simulink model "Final_3"  (R2022b)
settings: Solver=VariableStepAuto  StartTime=0.0  StopTime=20  RelTol=1e-3
libraries: cstblocks x22
settings Model: Creator=asus  LastModifiedBy=asus

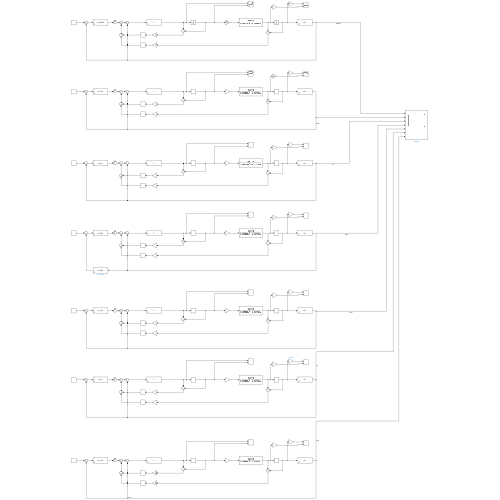
[thumbnail: Simulink's stored preview of the top-level diagram]
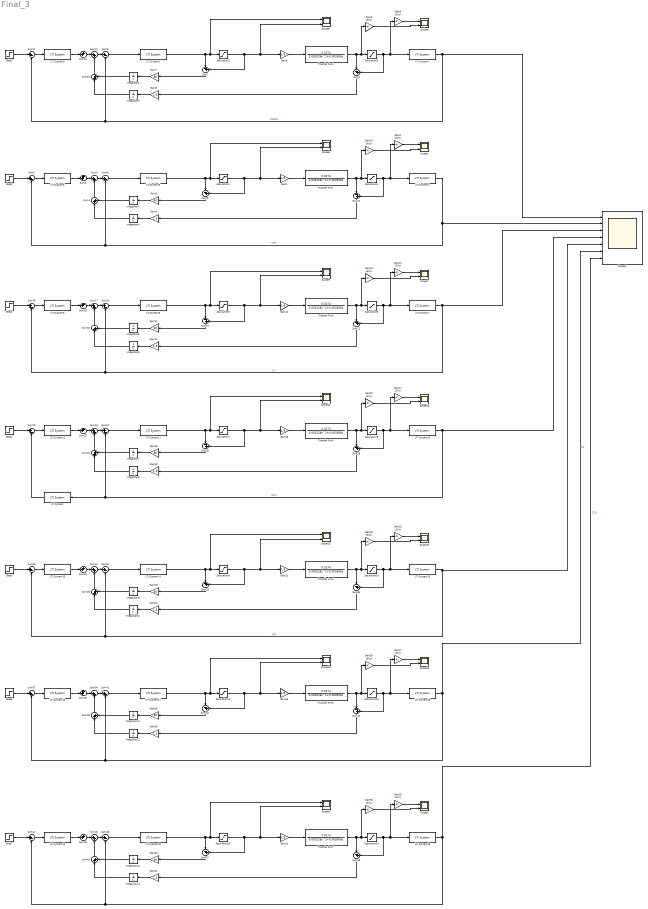
== system Final_3 ==
  Gain{1,5,11,16,21,26,31} (7 alike) : Gain  Gain=1/5
  Gain{2,6,9..10,12,15,17,20,22,25,27,30,32,35} (14 alike) : Gain  Gain=180/pi
  Gain{3,7,13,18,23,28,33} (7 alike) : Gain  Gain=80
  Gain{4,8,14,19,24,29,34} (7 alike) : Gain  Gain=1.5
  Integrator{1..14} (14 alike) : Integrator
  LTI System : cstblocks/LTI System  sys=H_RZN  IC=[]
  LTI System{1,4,7,10,13,16,19} (7 alike) : cstblocks/LTI System  sys=Gb  IC=[]
  LTI System{2,5,8,11,14,17,20} (7 alike) : cstblocks/LTI System  sys=C  IC=[]
  LTI System12 : cstblocks/LTI System  sys=G_RZN  IC=[]
  LTI System15 : cstblocks/LTI System  sys=G_WJC  IC=[]
  LTI System18 : cstblocks/LTI System  sys=G_CC  IC=[]
  LTI System21 : cstblocks/LTI System  sys=G_CCR  IC=[]
  LTI System3 : cstblocks/LTI System  sys=G_CHR20  IC=[]
  LTI System6 : cstblocks/LTI System  sys=G_CHR  IC=[]
  LTI System9 : cstblocks/LTI System  sys=G_ZN  IC=[]
  Saturation{1..2,5,7,9,11,13} (7 alike) : Saturate  UpperLimit=30  LowerLimit=-30
  Saturation{3..4,6,8,10,12,14} (7 alike) : Saturate  UpperLimit=pi*0.47  LowerLimit=-pi*0.47
  Scope{1..3,5..10,12..13,15..16,18} (14 alike) : Scope  NumInputPorts=2
  Scope4 : Scope  NumInputPorts=7
  Step{1..7} (7 alike) : Step  Time=0  After=1.5  SampleTime=0
  Sum{1,3,10,12,15,17,22,24,29,31,36,38,43,45} (14 alike) : Sum  Inputs=|++
  Sum{2,6,8,11,16,20,23,27,30,34,37,41,44,48} (14 alike) : Sum  Inputs=|+-
  Sum{4,13,18,25,32,39,46} (7 alike) : Sum  Inputs=++|
  Sum{5,7,9,14,19,21,26,28,33,35,40,42,47,49} (14 alike) : Sum  Inputs=|-+
  Transfer Fcn{1..7} (7 alike) : TransferFcn  Numerator=[0.0274]  Denominator=[0.003228 0.003508 0]
  wires:
  Gain5/1 -> Transfer Fcn3/1
  Gain7/1 -> Integrator2/1
  Sum11/1 -> LTI System3/1
  Saturation3/1 -> Sum9/2, LTI System1/1, Gain6/1
  LTI System1/1 -> Sum8/2, Sum11/2, Scope4/1  "CHR20"
  Saturation2/1 -> Sum7/2, Scope5/2, Gain5/1
  Transfer Fcn3/1 -> Gain9/1, Saturation3/1, Sum9/1
  Sum7/1 -> Gain7/1
  Integrator2/1 -> Sum10/2
  LTI System2/1 -> Scope5/1, Saturation2/1, Sum7/1
  Sum13/1 -> Sum12/1
  Sum8/1 -> LTI System2/1
  Step1/1 -> Sum11/1
  Gain6/1 -> Scope3/1
  Gain9/1 -> Scope3/2
  LTI System3/1 -> Sum13/2
  Gain8/1 -> Integrator3/1
  Sum12/1 -> Sum8/1
  Sum10/1 -> Sum12/2
  Sum9/1 -> Gain8/1
  Integrator3/1 -> Sum10/1
  Gain2/1 -> Scope1/1
  LTI System6/1 -> Sum4/2
  Sum1/1 -> Sum3/2
  Sum14/1 -> Gain4/1
  Gain1/1 -> Transfer Fcn1/1
  Transfer Fcn1/1 -> Gain10/1, Saturation4/1, Sum14/1
  Sum4/1 -> Sum3/1
  Gain4/1 -> Integrator4/1
  Step2/1 -> Sum2/1
  Integrator1/1 -> Sum1/2
  Saturation1/1 -> Sum5/2, Scope6/2, Gain1/1
  Gain3/1 -> Integrator1/1
  Saturation4/1 -> Sum14/2, LTI System4/1, Gain2/1
  Gain10/1 -> Scope1/2
  Sum2/1 -> LTI System6/1
  Sum5/1 -> Gain3/1
  Sum6/1 -> LTI System5/1
  LTI System4/1 -> Sum6/2, Sum2/2, Scope4/2  "CHR"
  LTI System5/1 -> Scope6/1, Saturation1/1, Sum5/1
  Integrator4/1 -> Sum1/1
  Sum3/1 -> Sum6/1
  Gain12/1 -> Scope7/1
  LTI System9/1 -> Sum18/2
  Sum15/1 -> Sum17/2
  Sum21/1 -> Gain14/1
  Gain11/1 -> Transfer Fcn2/1
  Transfer Fcn2/1 -> Gain15/1, Saturation6/1, Sum21/1
  Sum18/1 -> Sum17/1
  Gain14/1 -> Integrator6/1
  Step3/1 -> Sum16/1
  Integrator5/1 -> Sum15/2
  Saturation5/1 -> Sum19/2, Scope9/2, Gain11/1
  Gain13/1 -> Integrator5/1
  Saturation6/1 -> Sum21/2, LTI System7/1, Gain12/1
  Gain15/1 -> Scope7/2
  Sum16/1 -> LTI System9/1
  Sum19/1 -> Gain13/1
  Sum20/1 -> LTI System8/1
  LTI System7/1 -> Scope4/3, Sum20/2, Sum16/2  "ZN"
  LTI System8/1 -> Scope9/1, Saturation5/1, Sum19/1
  Integrator6/1 -> Sum15/1
  Sum17/1 -> Sum20/1
  Gain17/1 -> Scope10/1
  LTI System12/1 -> Sum25/2
  Sum22/1 -> Sum24/2
  Sum28/1 -> Gain19/1
  Gain16/1 -> Transfer Fcn4/1
  Transfer Fcn4/1 -> Gain20/1, Saturation8/1, Sum28/1
  Sum25/1 -> Sum24/1
  Gain19/1 -> Integrator8/1
  Step4/1 -> Sum23/1
  Integrator7/1 -> Sum22/2
  Saturation7/1 -> Sum26/2, Scope12/2, Gain16/1
  Gain18/1 -> Integrator7/1
  Saturation8/1 -> Sum28/2, LTI System10/1, Gain17/1
  Gain20/1 -> Scope10/2
  Sum23/1 -> LTI System12/1
  Sum26/1 -> Gain18/1
  Sum27/1 -> LTI System11/1
  LTI System10/1 -> Scope4/4, Sum27/2, LTI System/1  "RZN"
  LTI System11/1 -> Scope12/1, Saturation7/1, Sum26/1
  Integrator8/1 -> Sum22/1
  Sum24/1 -> Sum27/1
  Gain22/1 -> Scope13/1
  LTI System15/1 -> Sum32/2
  Sum29/1 -> Sum31/2
  Sum35/1 -> Gain24/1
  Gain21/1 -> Transfer Fcn5/1
  Transfer Fcn5/1 -> Gain25/1, Saturation10/1, Sum35/1
  Sum32/1 -> Sum31/1
  Gain24/1 -> Integrator10/1
  Step5/1 -> Sum30/1
  Integrator9/1 -> Sum29/2
  Saturation9/1 -> Sum33/2, Scope15/2, Gain21/1
  Gain23/1 -> Integrator9/1
  Saturation10/1 -> Sum35/2, LTI System13/1, Gain22/1
  Gain25/1 -> Scope13/2
  Sum30/1 -> LTI System15/1
  Sum33/1 -> Gain23/1
  Sum34/1 -> LTI System14/1
  LTI System13/1 -> Sum34/2, Sum30/2, Scope4/5  "WJC"
  LTI System14/1 -> Scope15/1, Saturation9/1, Sum33/1
  Integrator10/1 -> Sum29/1
  Sum31/1 -> Sum34/1
  Gain27/1 -> Scope16/1
  LTI System18/1 -> Sum39/2
  Sum36/1 -> Sum38/2
  Sum42/1 -> Gain29/1
  Gain26/1 -> Transfer Fcn6/1
  Transfer Fcn6/1 -> Gain30/1, Saturation12/1, Sum42/1
  Sum39/1 -> Sum38/1
  Gain29/1 -> Integrator12/1
  Step6/1 -> Sum37/1
  Integrator11/1 -> Sum36/2
  Saturation11/1 -> Sum40/2, Scope18/2, Gain26/1
  Gain28/1 -> Integrator11/1
  Saturation12/1 -> Sum42/2, LTI System16/1, Gain27/1
  Gain30/1 -> Scope16/2
  Sum37/1 -> LTI System18/1
  Sum40/1 -> Gain28/1
  Sum41/1 -> LTI System17/1
  LTI System16/1 -> Scope4/6, Sum41/2, Sum37/2  "CC"
  LTI System17/1 -> Scope18/1, Saturation11/1, Sum40/1
  Integrator12/1 -> Sum36/1
  Sum38/1 -> Sum41/1
  LTI System/1 -> Sum23/2
  Sum45/1 -> Sum48/1
  Integrator14/1 -> Sum43/1
  LTI System20/1 -> Scope8/1, Saturation13/1, Sum47/1
  Sum48/1 -> LTI System20/1
  Sum47/1 -> Gain33/1
  Saturation14/1 -> Sum49/2, LTI System19/1, Gain32/1
  Saturation13/1 -> Sum47/2, Scope8/2, Gain31/1
  Gain33/1 -> Integrator13/1
  Gain34/1 -> Integrator14/1
  Step7/1 -> Sum44/1
  Transfer Fcn7/1 -> Gain35/1, Saturation14/1, Sum49/1
  Sum46/1 -> Sum45/1
  Integrator13/1 -> Sum43/2
  Gain35/1 -> Scope2/2
  LTI System19/1 -> Scope4/7, Sum48/2, Sum44/2  "CCR"
  Gain31/1 -> Transfer Fcn7/1
  Sum43/1 -> Sum45/2
  Sum49/1 -> Gain34/1
  LTI System21/1 -> Sum46/2
  Sum44/1 -> LTI System21/1
  Gain32/1 -> Scope2/1
